simulink model "BicycleHome"  (R2017b)
settings: Solver=VariableStepAuto  StartTime=0.0  StopTime=100  RelTol=1e-3
values from neighbouring files (symbols this model uses):
  b_contact_FW = 2e3    (= 2000)    [BicycleInit.m]
  b_contact_RW = 2e3    (= 2000)    [BicycleInit.m]
  C_F_alpha = 2e4    (= 20000)    [BicycleInit.m]
  C_F_kappa = 2e4    (= 20000)    [BicycleInit.m]
  CM_phi = 1e-1    (= 0.1)    [BicycleInit.m]
  Dtheta0 = -v0 / radiusRW    (= -24.3333333333)    [BicycleInit.m]
  Dtheta0_FW = -v0 / radiusFW    (= -20.8571428571)    [BicycleInit.m]
  epsilon = 1e-2    (= 0.01)    [BicycleInit.m]
  g = 9.81    [BicycleInit.m]
  k_contact_FW = 1e6    (= 1000000)    [BicycleInit.m]
  k_contact_RW = 1e6    (= 1000000)    [BicycleInit.m]
  lengthFF = frontHinge / (sind(lambda))    [BicycleInit.m]
  lengthFW = 0.03    [BicycleInit.m]
  lengthRF = sqrt((w-frontHinge)^2 + adj^2)    [BicycleInit.m]
  lengthRW = 0.03    [BicycleInit.m]
  massFW = 4    [BicycleInit.m]
  massRW = 2    [BicycleInit.m]
  mB = 85    [BicycleInit.m]
  mH = 5    [BicycleInit.m]
  radiusFW = 0.35    [BicycleInit.m]
  radiusRW = 0.3    [BicycleInit.m]
  sigma = 0.12    [BicycleInit.m]
  xPla = 25    [BicycleInit.m]
  yPla = 15    [BicycleInit.m]
  zPla = 0.01    [BicycleInit.m]
undefined symbols (not defined in the file or in its folder): Cylinder, Parts_Lib, sigbuilder_block, X, Y, Z
libraries: nesl_utility x43, sm_lib x37, vrlib x21, dspsrcs4 x2, simulink x2
(part 2 of 3)

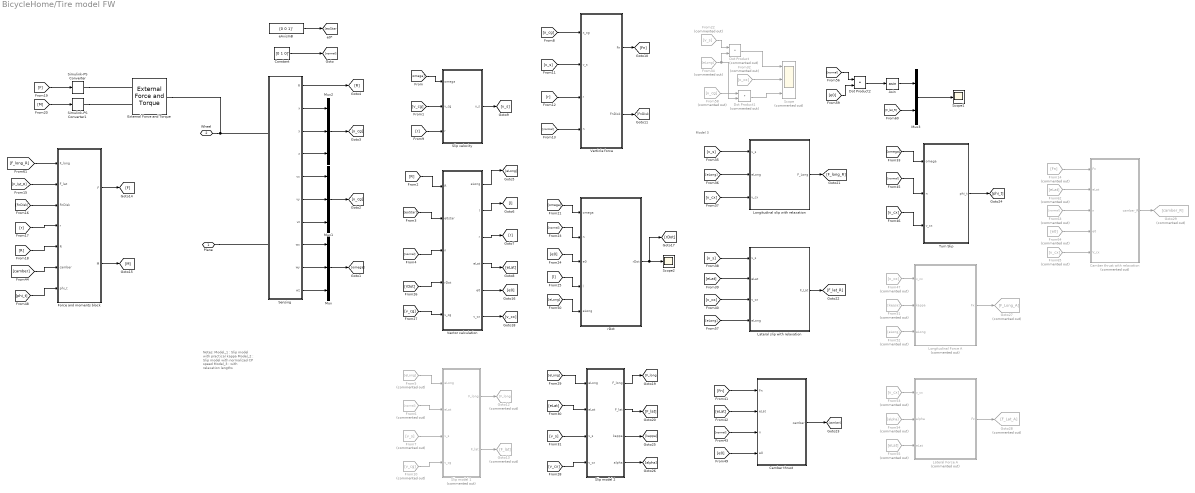
== system BicycleHome/Tire model FW ==
  note: Model 3
  note: Notes:
      | Model_1 : Slip model with practical kappa
      | Model_2 : Slip model with normalized CP speed
      | Model_3 : with relaxation lengths
  Asin : Trigonometry  Operator=asin
  Camber thrust : Subsystem
  Camber thrust with relaxation : Subsystem  Commented=on
  Constant : Constant  Value=[0 1 0]'
  Dot Product : DotProduct  Commented=on  InputSameDT=on  OutDataTypeStr=Inherit: Inherit via internal rule
  Dot Product1 : DotProduct  Commented=on  InputSameDT=on  OutDataTypeStr=Inherit: Inherit via internal rule
  Dot Product2 : DotProduct  InputSameDT=on  OutDataTypeStr=Inherit: Inherit via internal rule
  External Force and Torque : sm_lib/Forces and Torques/External Force and Torque  ForceResolutionFrame=AttachedFrame  EnableForceX=off  EnableForceY=off  EnableForceZ=off  EnableForce=on  TorqueResolutionFrame=AttachedFrame  EnableTorqueX=off  EnableTorqueY=off  EnableTorqueZ=off  EnableTorque=on
  Force and moments block : Subsystem
  From10 : From  Commented=on  GotoTag=v_cg
  From14 : From  Commented=on  GotoTag=Fn
  From22 : From  Commented=on  GotoTag=v_s
  From{32,47,53,65} (4 alike) : From  Commented=on  GotoTag=v_cx
  From34 : From  Commented=on  GotoTag=eLong
  From5 : From  Commented=on  GotoTag=eLong
  From51 : From  Commented=on  GotoTag=kappa
  From52 : From  Commented=on  GotoTag=eLong
  From54 : From  Commented=on  GotoTag=alpha
  From55 : From  Commented=on  GotoTag=eLat
  From58 : From  Commented=on  GotoTag=v_cg
  From6 : From  Commented=on  GotoTag=normal
  From62 : From  Commented=on  GotoTag=eLat
  From63 : From  Commented=on  GotoTag=normal
  From64 : From  Commented=on  GotoTag=e0
  From7 : From  Commented=on  GotoTag=v_s
  Goto12 : Goto  Commented=on  GotoTag=F_long
  Goto13 : Goto  Commented=on  GotoTag=F_lat
  Goto27 : Goto  Commented=on  GotoTag=F_Long_A
  Goto28 : Goto  Commented=on  GotoTag=F_Lat_A
  Goto29 : Goto  Commented=on  GotoTag=camber_R
  Lateral Force A : Subsystem  Commented=on
  Lateral slip with relaxation : Subsystem
  Longitudinal Force A : Subsystem  Commented=on
  Longitudinal slip with relaxation : Subsystem
  Mux : Mux  Inputs=3
  Mux1 : Mux  Inputs=3
  Mux2 : Mux  Inputs=3
  Mux3 : Mux  Inputs=2
  Scope : Scope  Commented=on  NumInputPorts=3
  Scope1 : Scope
  Scope2 : Scope
  Sensing : Subsystem
  Simulink-PS Converter : nesl_utility/Simulink-PS Converter  PhysicalDomain=network_engine_domain  SubClassName=ps_input  LeftPortType=input  RightPortType=output  PseudoPeriodic=off  Frequencies=[]  NoiseDistribution=none  NoiseParameters=[]  Unit=N  AffineConversion=off  FilteringAndDerivatives=provide  SimscapeFilterOrder=1  InputFilterTimeConstant=0.001  UdotUserProvided=0
  Simulink-PS Converter1 : nesl_utility/Simulink-PS Converter  PhysicalDomain=network_engine_domain  SubClassName=ps_input  LeftPortType=input  RightPortType=output  PseudoPeriodic=off  Frequencies=[]  NoiseDistribution=none  NoiseParameters=[]  Unit=N*m  AffineConversion=off  FilteringAndDerivatives=provide  SimscapeFilterOrder=1  InputFilterTimeConstant=0.001  UdotUserProvided=0
  Slip model 1 : Subsystem  Commented=on
  Slip model 2 : Subsystem
  Slip velocity : Subsystem
  Turn Slip : Subsystem
  Vector calculation : Subsystem
  Verticle force : Subsystem
  eAxisInB : Constant  Value=[0 0 1]'
  rDot : Subsystem
  Plane : PMIOPort  Port=1  Side=Left
  Wheel : PMIOPort  Port=2  Side=Right
  wires:
  eAxisInB/1 -> [eoStar]
  Constant/1 -> [normal]
  Sensing/8(wx) -> Mux/1
  Sensing/9(wy) -> Mux/2
  Sensing/10(wz) -> Mux/3
  Mux/1 -> [omega]
  [omega] -> Slip velocity/1(omega)
  Sensing/5(vx) -> Mux1/1
  Sensing/6(vy) -> Mux1/2
  Sensing/7(vz) -> Mux1/3
  Mux1/1 -> [v_cg]
  [v_cg] -> Slip velocity/2(v_cg)
  Sensing/2(x) -> Mux2/1
  Sensing/3(y) -> Mux2/2
  Sensing/4(z) -> Mux2/3
  Mux2/1 -> [x_cg]
  Sensing/1(R) -> [R]
  [R] -> Vector calculation/1(R)
  [eoStar] -> Vector calculation/2(e0star)
  [normal] -> Vector calculation/3(n)
  From5/1 -> Slip model 1/1(eLong)
  From6/1 -> Slip model 1/2(eLat)
  Vector calculation/1(eLong) -> [eLong]
  Vector calculation/2(l) -> [l]
  Vector calculation/3(r) -> [r]
  Vector calculation/4(eLat) -> [eLat]
  [r] -> Slip velocity/3(r)
  Slip velocity/1(v_s) -> [v_s]
  From7/1 -> Slip model 1/3(v_s)
  From10/1 -> Slip model 1/4(v_cg)
  [x_cg] -> Verticle force/1(x_cg)
  [v_s] -> Verticle force/2(v_s)
  [r] -> Verticle force/3(r)
  [normal] -> Verticle force/4(n)
  Verticle force/1(Fn) -> [Fn]
  Verticle force/2(FnDisk) -> [FnDisk]
  Slip model 1/1(F_long) -> Goto12/1
  Slip model 1/2(F_lat) -> Goto13/1
  [r] -> Force and moments block/4(r)
  [R] -> Force and moments block/5(R)
  [F] -> Simulink-PS Converter/1
  [M] -> Simulink-PS Converter1/1
  Vector calculation/5(e0) -> [e0]
  [v_cg] -> Vector calculation/5(v_cg)
  Vector calculation/6(v_cx) -> [v_cx]
  Slip model 2/1(F_long) -> [F_long]
  [v_s] -> Slip model 2/3(v_s)
  [eLat] -> Slip model 2/2(eLat)
  [eLong] -> Slip model 2/1(eLong)
  Slip model 2/2(F_lat) -> [F_lat]
  [v_cx] -> Slip model 2/4(v_cx)
  From22/1 -> Dot Product/1
  From34/1 -> Dot Product1/2, Dot Product/2
  Dot Product/1 -> Scope/1
  [v_s] -> Longitudinal slip with relaxation/1(v_s)
  [eLong] -> Longitudinal slip with relaxation/2(eLong)
  [v_cx] -> Longitudinal slip with relaxation/3(v_cx)
  Longitudinal slip with relaxation/1(F_Long) -> [F_long_R]
  [eLat] -> Lateral slip with relaxation/2(eLat)
  Lateral slip with relaxation/1(F_Lat) -> [F_lat_R]
  [v_cx] -> Lateral slip with relaxation/3(v_cx)
  [v_s] -> Lateral slip with relaxation/1(v_s)
  [Fn] -> Camber thrust/1(Fn)
  [eLat] -> Camber thrust/2(eLat)
  [normal] -> Camber thrust/3(n)
  Camber thrust/1(camber) -> [camber]
  [e0] -> Camber thrust/4(e0)
  Force and moments block/1(F) -> [F]
  Force and moments block/2(M) -> [M]
  [eLong] -> Lateral slip with relaxation/4(eLong)
  From32/1 -> Scope/2
  From58/1 -> Dot Product1/1
  Dot Product1/1 -> Scope/3
  [omega] -> rDot/1(omega)
  [normal] -> rDot/2(n)
  [e0] -> rDot/3(e0)
  [l] -> rDot/4(l)
  [eLong] -> rDot/5(eLong)
  rDot/1(rDot) -> [rDot], Scope2/1
  [rDot] -> Vector calculation/4(rDot)
  Slip model 2/3(kappa) -> [kappa]
  [omega] -> Turn Slip/1(omega)
  [normal] -> Turn Slip/2(n)
  [v_cx] -> Turn Slip/3(v_cx)
  Turn Slip/1(phi_t) -> [phi_t]
  From47/1 -> Longitudinal Force A/1(v_cx)
  Slip model 2/4(alpha) -> [alpha]
  From51/1 -> Longitudinal Force A/2(kappa)
  From52/1 -> Longitudinal Force A/3(eLong)
  Longitudinal Force A/1(Fx) -> Goto27/1
  From53/1 -> Lateral Force A/1(v_cx)
  From54/1 -> Lateral Force A/2(alpha)
  From55/1 -> Lateral Force A/3(eLat)
  Lateral Force A/1(Fz) -> Goto28/1
  [normal] -> Dot Product2/1
  [e0] -> Dot Product2/2
  Dot Product2/1 -> Asin/1
  Asin/1 -> Mux3/1
  [F_lat_R] -> Mux3/2
  Mux3/1 -> Scope1/1
  [FnDisk] -> Force and moments block/3(FnDisk)
  [camber] -> Force and moments block/6(camber)
  [F_long_R] -> Force and moments block/1(F_long)
  [F_lat_R] -> Force and moments block/2(F_lat)
  From62/1 -> Camber thrust with relaxation/2(eLat)
  From64/1 -> Camber thrust with relaxation/4(e0)
  From63/1 -> Camber thrust with relaxation/3(n)
  From14/1 -> Camber thrust with relaxation/1(Fn)
  From65/1 -> Camber thrust with relaxation/5(V_cx)
  Camber thrust with relaxation/1(camber_R) -> Goto29/1
  [phi_t] -> Force and moments block/7(phi_t)
  connections:
  Plane/RConn1 -- Sensing/LConn2
  Wheel/RConn1 -- External Force and Torque/RConn1 -- Sensing/LConn1
  Simulink-PS Converter/RConn1 -- External Force and Torque/LConn1
  Simulink-PS Converter1/RConn1 -- External Force and Torque/LConn2

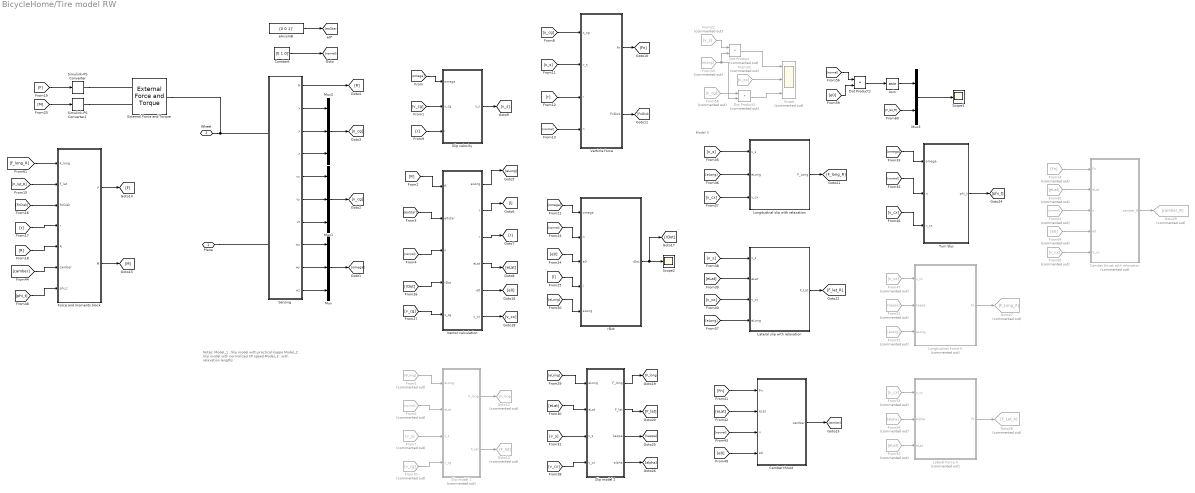
== system BicycleHome/Tire model RW ==
  note: Model 3
  note: Notes:
      | Model_1 : Slip model with practical kappa
      | Model_2 : Slip model with normalized CP speed
      | Model_3 : with relaxation lengths
  Asin : Trigonometry  Operator=asin
  Camber thrust : Subsystem
  Camber thrust with relaxation : Subsystem  Commented=on
  Constant : Constant  Value=[0 1 0]'
  Dot Product : DotProduct  Commented=on  InputSameDT=on  OutDataTypeStr=Inherit: Inherit via internal rule
  Dot Product1 : DotProduct  Commented=on  InputSameDT=on  OutDataTypeStr=Inherit: Inherit via internal rule
  Dot Product2 : DotProduct  InputSameDT=on  OutDataTypeStr=Inherit: Inherit via internal rule
  External Force and Torque : sm_lib/Forces and Torques/External Force and Torque  ForceResolutionFrame=AttachedFrame  EnableForceX=off  EnableForceY=off  EnableForceZ=off  EnableForce=on  TorqueResolutionFrame=AttachedFrame  EnableTorqueX=off  EnableTorqueY=off  EnableTorqueZ=off  EnableTorque=on
  Force and moments block : Subsystem
  From10 : From  Commented=on  GotoTag=v_cg
  From14 : From  Commented=on  GotoTag=Fn
  From22 : From  Commented=on  GotoTag=v_s
  From{32,47,53,65} (4 alike) : From  Commented=on  GotoTag=v_cx
  From34 : From  Commented=on  GotoTag=eLong
  From5 : From  Commented=on  GotoTag=eLong
  From51 : From  Commented=on  GotoTag=kappa
  From52 : From  Commented=on  GotoTag=eLong
  From54 : From  Commented=on  GotoTag=alpha
  From55 : From  Commented=on  GotoTag=eLat
  From58 : From  Commented=on  GotoTag=v_cg
  From6 : From  Commented=on  GotoTag=normal
  From62 : From  Commented=on  GotoTag=eLat
  From63 : From  Commented=on  GotoTag=normal
  From64 : From  Commented=on  GotoTag=e0
  From7 : From  Commented=on  GotoTag=v_s
  Goto12 : Goto  Commented=on  GotoTag=F_long
  Goto13 : Goto  Commented=on  GotoTag=F_lat
  Goto27 : Goto  Commented=on  GotoTag=F_Long_A
  Goto28 : Goto  Commented=on  GotoTag=F_Lat_A
  Goto29 : Goto  Commented=on  GotoTag=camber_R
  Lateral Force A : Subsystem  Commented=on
  Lateral slip with relaxation : Subsystem
  Longitudinal Force A : Subsystem  Commented=on
  Longitudinal slip with relaxation : Subsystem
  Mux : Mux  Inputs=3
  Mux1 : Mux  Inputs=3
  Mux2 : Mux  Inputs=3
  Mux3 : Mux  Inputs=2
  Scope : Scope  Commented=on  NumInputPorts=3
  Scope1 : Scope
  Scope2 : Scope
  Sensing : Subsystem
  Simulink-PS Converter : nesl_utility/Simulink-PS Converter  PhysicalDomain=network_engine_domain  SubClassName=ps_input  LeftPortType=input  RightPortType=output  PseudoPeriodic=off  Frequencies=[]  NoiseDistribution=none  NoiseParameters=[]  Unit=N  AffineConversion=off  FilteringAndDerivatives=provide  SimscapeFilterOrder=1  InputFilterTimeConstant=0.001  UdotUserProvided=0
  Simulink-PS Converter1 : nesl_utility/Simulink-PS Converter  PhysicalDomain=network_engine_domain  SubClassName=ps_input  LeftPortType=input  RightPortType=output  PseudoPeriodic=off  Frequencies=[]  NoiseDistribution=none  NoiseParameters=[]  Unit=N*m  AffineConversion=off  FilteringAndDerivatives=provide  SimscapeFilterOrder=1  InputFilterTimeConstant=0.001  UdotUserProvided=0
  Slip model 1 : Subsystem  Commented=on
  Slip model 2 : Subsystem
  Slip velocity : Subsystem
  Turn Slip : Subsystem
  Vector calculation : Subsystem
  Verticle force : Subsystem
  eAxisInB : Constant  Value=[0 0 1]'
  rDot : Subsystem
  Plane : PMIOPort  Port=1  Side=Left
  Wheel : PMIOPort  Port=2  Side=Right
  wires:
  eAxisInB/1 -> [eoStar]
  Constant/1 -> [normal]
  Sensing/8(wx) -> Mux/1
  Sensing/9(wy) -> Mux/2
  Sensing/10(wz) -> Mux/3
  Mux/1 -> [omega]
  [omega] -> Slip velocity/1(omega)
  Sensing/5(vx) -> Mux1/1
  Sensing/6(vy) -> Mux1/2
  Sensing/7(vz) -> Mux1/3
  Mux1/1 -> [v_cg]
  [v_cg] -> Slip velocity/2(v_cg)
  Sensing/2(x) -> Mux2/1
  Sensing/3(y) -> Mux2/2
  Sensing/4(z) -> Mux2/3
  Mux2/1 -> [x_cg]
  Sensing/1(R) -> [R]
  [R] -> Vector calculation/1(R)
  [eoStar] -> Vector calculation/2(e0star)
  [normal] -> Vector calculation/3(n)
  From5/1 -> Slip model 1/1(eLong)
  From6/1 -> Slip model 1/2(eLat)
  Vector calculation/1(eLong) -> [eLong]
  Vector calculation/2(l) -> [l]
  Vector calculation/3(r) -> [r]
  Vector calculation/4(eLat) -> [eLat]
  [r] -> Slip velocity/3(r)
  Slip velocity/1(v_s) -> [v_s]
  From7/1 -> Slip model 1/3(v_s)
  From10/1 -> Slip model 1/4(v_cg)
  [x_cg] -> Verticle force/1(x_cg)
  [v_s] -> Verticle force/2(v_s)
  [r] -> Verticle force/3(r)
  [normal] -> Verticle force/4(n)
  Verticle force/1(Fn) -> [Fn]
  Verticle force/2(FnDisk) -> [FnDisk]
  Slip model 1/1(F_long) -> Goto12/1
  Slip model 1/2(F_lat) -> Goto13/1
  [r] -> Force and moments block/4(r)
  [R] -> Force and moments block/5(R)
  [F] -> Simulink-PS Converter/1
  [M] -> Simulink-PS Converter1/1
  Vector calculation/5(e0) -> [e0]
  [v_cg] -> Vector calculation/5(v_cg)
  Vector calculation/6(v_cx) -> [v_cx]
  Slip model 2/1(F_long) -> [F_long]
  [v_s] -> Slip model 2/3(v_s)
  [eLat] -> Slip model 2/2(eLat)
  [eLong] -> Slip model 2/1(eLong)
  Slip model 2/2(F_lat) -> [F_lat]
  [v_cx] -> Slip model 2/4(v_cx)
  From22/1 -> Dot Product/1
  From34/1 -> Dot Product1/2, Dot Product/2
  Dot Product/1 -> Scope/1
  [v_s] -> Longitudinal slip with relaxation/1(v_s)
  [eLong] -> Longitudinal slip with relaxation/2(eLong)
  [v_cx] -> Longitudinal slip with relaxation/3(v_cx)
  Longitudinal slip with relaxation/1(F_Long) -> [F_long_R]
  [eLat] -> Lateral slip with relaxation/2(eLat)
  Lateral slip with relaxation/1(F_Lat) -> [F_lat_R]
  [v_cx] -> Lateral slip with relaxation/3(v_cx)
  [v_s] -> Lateral slip with relaxation/1(v_s)
  [Fn] -> Camber thrust/1(Fn)
  [eLat] -> Camber thrust/2(eLat)
  [normal] -> Camber thrust/3(n)
  Camber thrust/1(camber) -> [camber]
  [e0] -> Camber thrust/4(e0)
  Force and moments block/1(F) -> [F]
  Force and moments block/2(M) -> [M]
  [eLong] -> Lateral slip with relaxation/4(eLong)
  From32/1 -> Scope/2
  From58/1 -> Dot Product1/1
  Dot Product1/1 -> Scope/3
  [omega] -> rDot/1(omega)
  [normal] -> rDot/2(n)
  [e0] -> rDot/3(e0)
  [l] -> rDot/4(l)
  [eLong] -> rDot/5(eLong)
  rDot/1(rDot) -> [rDot], Scope2/1
  [rDot] -> Vector calculation/4(rDot)
  Slip model 2/3(kappa) -> [kappa]
  [omega] -> Turn Slip/1(omega)
  [normal] -> Turn Slip/2(n)
  [v_cx] -> Turn Slip/3(v_cx)
  Turn Slip/1(phi_t) -> [phi_t]
  From47/1 -> Longitudinal Force A/1(v_cx)
  Slip model 2/4(alpha) -> [alpha]
  From51/1 -> Longitudinal Force A/2(kappa)
  From52/1 -> Longitudinal Force A/3(eLong)
  Longitudinal Force A/1(Fx) -> Goto27/1
  From53/1 -> Lateral Force A/1(v_cx)
  From54/1 -> Lateral Force A/2(alpha)
  From55/1 -> Lateral Force A/3(eLat)
  Lateral Force A/1(Fz) -> Goto28/1
  [normal] -> Dot Product2/1
  [e0] -> Dot Product2/2
  Dot Product2/1 -> Asin/1
  Asin/1 -> Mux3/1
  [F_lat_R] -> Mux3/2
  Mux3/1 -> Scope1/1
  [FnDisk] -> Force and moments block/3(FnDisk)
  [camber] -> Force and moments block/6(camber)
  [F_long_R] -> Force and moments block/1(F_long)
  [F_lat_R] -> Force and moments block/2(F_lat)
  From62/1 -> Camber thrust with relaxation/2(eLat)
  From64/1 -> Camber thrust with relaxation/4(e0)
  From63/1 -> Camber thrust with relaxation/3(n)
  From14/1 -> Camber thrust with relaxation/1(Fn)
  From65/1 -> Camber thrust with relaxation/5(V_cx)
  Camber thrust with relaxation/1(camber_R) -> Goto29/1
  [phi_t] -> Force and moments block/7(phi_t)
  connections:
  Plane/RConn1 -- Sensing/LConn2
  Wheel/RConn1 -- External Force and Torque/RConn1 -- Sensing/LConn1
  Simulink-PS Converter/RConn1 -- External Force and Torque/LConn1
  Simulink-PS Converter1/RConn1 -- External Force and Torque/LConn2

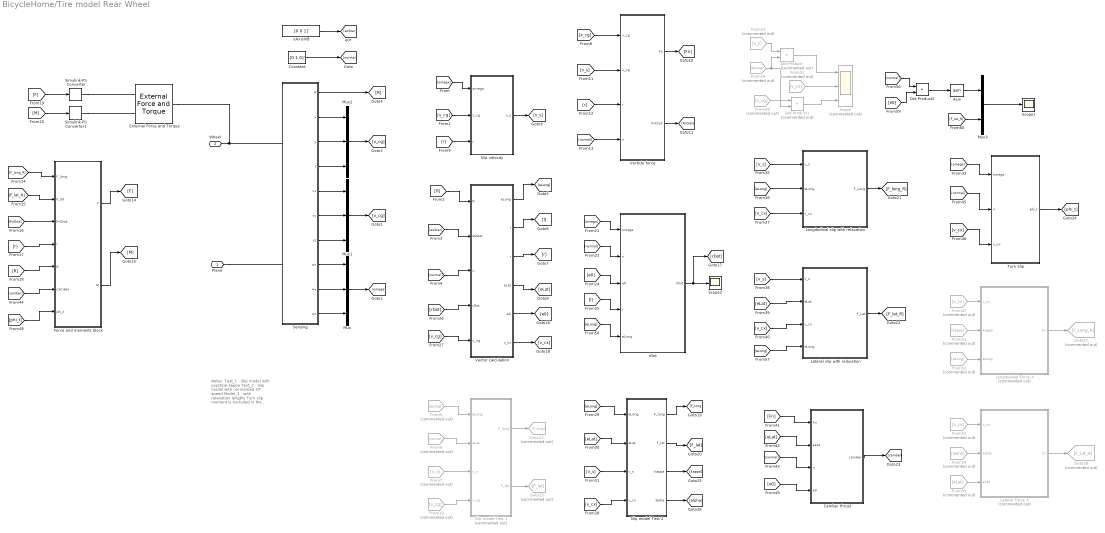
== system BicycleHome/Tire model Rear Wheel ==
  note: Notes:
      | Test_1 : Slip model with practical kappa
      | Test_2 : Slip model with normalized CP speed
      | Model_3 : with relaxation lengths
      |
      | Turn slip moment is excluded in the model as per the
      | paper by RS Sharp
  Asin : Trigonometry  Operator=asin
  Camber thrust : Subsystem
  Constant : Constant  Value=[0 1 0]'
  Dot Product : DotProduct  Commented=on  InputSameDT=on  OutDataTypeStr=Inherit: Inherit via internal rule
  Dot Product1 : DotProduct  Commented=on  InputSameDT=on  OutDataTypeStr=Inherit: Inherit via internal rule
  Dot Product2 : DotProduct  InputSameDT=on  OutDataTypeStr=Inherit: Inherit via internal rule
  External Force and Torque : sm_lib/Forces and Torques/External Force and Torque  ForceResolutionFrame=AttachedFrame  EnableForceX=off  EnableForceY=off  EnableForceZ=off  EnableForce=on  TorqueResolutionFrame=AttachedFrame  EnableTorqueX=off  EnableTorqueY=off  EnableTorqueZ=off  EnableTorque=on
  Force and moments block : Subsystem
  From10 : From  Commented=on  GotoTag=v_cg
  From22 : From  Commented=on  GotoTag=v_s
  From32 : From  Commented=on  GotoTag=v_cx
  From34 : From  Commented=on  GotoTag=eLong
  From47 : From  Commented=on  GotoTag=v_cx
  From5 : From  Commented=on  GotoTag=eLong
  From51 : From  Commented=on  GotoTag=kappa
  From52 : From  Commented=on  GotoTag=eLong
  From53 : From  Commented=on  GotoTag=v_cx
  From54 : From  Commented=on  GotoTag=alpha
  From55 : From  Commented=on  GotoTag=eLat
  From58 : From  Commented=on  GotoTag=v_cg
  From6 : From  Commented=on  GotoTag=normal
  From7 : From  Commented=on  GotoTag=v_s
  Goto12 : Goto  Commented=on  GotoTag=F_long
  Goto13 : Goto  Commented=on  GotoTag=F_lat
  Goto27 : Goto  Commented=on  GotoTag=F_Long_A
  Goto28 : Goto  Commented=on  GotoTag=F_Lat_A
  Lateral Force A : Subsystem  Commented=on
  Lateral slip with relaxation : Subsystem
  Longitudinal Force A : Subsystem  Commented=on
  Longitudinal slip with relaxation : Subsystem
  Mux : Mux  Inputs=3
  Mux1 : Mux  Inputs=3
  Mux2 : Mux  Inputs=3
  Mux3 : Mux  Inputs=2
  Scope : Scope  Commented=on  NumInputPorts=3
  Scope1 : Scope
  Scope2 : Scope
  Sensing : Subsystem
  Simulink-PS Converter : nesl_utility/Simulink-PS Converter  PhysicalDomain=network_engine_domain  SubClassName=ps_input  LeftPortType=input  RightPortType=output  PseudoPeriodic=off  Frequencies=[]  NoiseDistribution=none  NoiseParameters=[]  Unit=N  AffineConversion=off  FilteringAndDerivatives=provide  SimscapeFilterOrder=1  InputFilterTimeConstant=0.001  UdotUserProvided=0
  Simulink-PS Converter1 : nesl_utility/Simulink-PS Converter  PhysicalDomain=network_engine_domain  SubClassName=ps_input  LeftPortType=input  RightPortType=output  PseudoPeriodic=off  Frequencies=[]  NoiseDistribution=none  NoiseParameters=[]  Unit=N*m  AffineConversion=off  FilteringAndDerivatives=provide  SimscapeFilterOrder=1  InputFilterTimeConstant=0.001  UdotUserProvided=0
  Slip model Test 1 : Subsystem  Commented=on
  Slip model Test 2 : Subsystem
  Slip velocity : Subsystem
  Turn Slip : Subsystem
  Vector calculation : Subsystem
  Verticle force : Subsystem
  eAxisInB : Constant  Value=[0 0 1]'
  rDot : Subsystem
  Plane : PMIOPort  Port=1  Side=Left
  Wheel : PMIOPort  Port=2  Side=Right
  wires:
  eAxisInB/1 -> [eoStar]
  Constant/1 -> [normal]
  Sensing/8(wx) -> Mux/1
  Sensing/9(wy) -> Mux/2
  Sensing/10(wz) -> Mux/3
  Mux/1 -> [omega]
  [omega] -> Slip velocity/1(omega)
  Sensing/5(vx) -> Mux1/1
  Sensing/6(vy) -> Mux1/2
  Sensing/7(vz) -> Mux1/3
  Mux1/1 -> [v_cg]
  [v_cg] -> Slip velocity/2(v_cg)
  Sensing/2(x) -> Mux2/1
  Sensing/3(y) -> Mux2/2
  Sensing/4(z) -> Mux2/3
  Mux2/1 -> [x_cg]
  Sensing/1(R) -> [R]
  [R] -> Vector calculation/1(R)
  [eoStar] -> Vector calculation/2(e0star)
  [normal] -> Vector calculation/3(n)
  From5/1 -> Slip model Test 1/1(eLong)
  From6/1 -> Slip model Test 1/2(eLat)
  Vector calculation/1(eLong) -> [eLong]
  Vector calculation/2(l) -> [l]
  Vector calculation/3(r) -> [r]
  Vector calculation/4(eLat) -> [eLat]
  [r] -> Slip velocity/3(r)
  Slip velocity/1(v_s) -> [v_s]
  From7/1 -> Slip model Test 1/3(v_s)
  From10/1 -> Slip model Test 1/4(v_cg)
  [x_cg] -> Verticle force/1(x_cg)
  [v_s] -> Verticle force/2(v_cg)
  [r] -> Verticle force/3(r)
  [normal] -> Verticle force/4(n)
  Verticle force/1(Fn) -> [Fn]
  Verticle force/2(FnDisk) -> [FnDisk]
  Slip model Test 1/1(F_long) -> Goto12/1
  Slip model Test 1/2(F_lat) -> Goto13/1
  [r] -> Force and moments block/4(r)
  [R] -> Force and moments block/5(R)
  [F] -> Simulink-PS Converter/1
  [M] -> Simulink-PS Converter1/1
  Vector calculation/5(e0) -> [e0]
  [v_cg] -> Vector calculation/5(v_cg)
  Vector calculation/6(v_cx) -> [v_cx]
  Slip model Test 2/1(F_long) -> [F_long]
  [v_s] -> Slip model Test 2/3(v_s)
  [eLat] -> Slip model Test 2/2(eLat)
  [eLong] -> Slip model Test 2/1(eLong)
  Slip model Test 2/2(F_lat) -> [F_lat]
  [v_cx] -> Slip model Test 2/4(v_cx)
  From22/1 -> Dot Product/1
  From34/1 -> Dot Product1/2, Dot Product/2
  Dot Product/1 -> Scope/1
  [v_s] -> Longitudinal slip with relaxation/1(v_s)
  [eLong] -> Longitudinal slip with relaxation/2(eLong)
  [v_cx] -> Longitudinal slip with relaxation/3(v_cx)
  Longitudinal slip with relaxation/1(F_Long) -> [F_long_R]
  [eLat] -> Lateral slip with relaxation/2(eLat)
  Lateral slip with relaxation/1(F_Lat) -> [F_lat_R]
  [v_cx] -> Lateral slip with relaxation/3(v_cx)
  [v_s] -> Lateral slip with relaxation/1(v_s)
  [Fn] -> Camber thrust/1(Fn)
  [eLat] -> Camber thrust/2(eLat)
  [normal] -> Camber thrust/3(n)
  Camber thrust/1(camber) -> [camber]
  [e0] -> Camber thrust/4(e0)
  Force and moments block/1(F) -> [F]
  Force and moments block/2(M) -> [M]
  [eLong] -> Lateral slip with relaxation/4(eLong)
  From32/1 -> Scope/2
  From58/1 -> Dot Product1/1
  Dot Product1/1 -> Scope/3
  [omega] -> rDot/1(omega)
  [normal] -> rDot/2(n)
  [e0] -> rDot/3(e0)
  [l] -> rDot/4(l)
  [eLong] -> rDot/5(eLong)
  rDot/1(rDot) -> [rDot], Scope2/1
  [rDot] -> Vector calculation/4(rDot)
  Slip model Test 2/3(kappa) -> [kappa]
  [omega] -> Turn Slip/1(omega)
  [normal] -> Turn Slip/2(n)
  [v_cx] -> Turn Slip/3(v_cx)
  Turn Slip/1(phi_t) -> [phi_t]
  From47/1 -> Longitudinal Force A/1(v_cx)
  Slip model Test 2/4(alpha) -> [alpha]
  From51/1 -> Longitudinal Force A/2(kappa)
  From52/1 -> Longitudinal Force A/3(eLong)
  Longitudinal Force A/1(Fx) -> Goto27/1
  From53/1 -> Lateral Force A/1(v_cx)
  From54/1 -> Lateral Force A/2(alpha)
  From55/1 -> Lateral Force A/3(eLat)
  Lateral Force A/1(Fz) -> Goto28/1
  [normal] -> Dot Product2/1
  [e0] -> Dot Product2/2
  Dot Product2/1 -> Asin/1
  Asin/1 -> Mux3/1
  [F_lat_R] -> Mux3/2
  Mux3/1 -> Scope1/1
  [FnDisk] -> Force and moments block/3(FnDisk)
  [F_long_R] -> Force and moments block/1(F_long)
  [F_lat_R] -> Force and moments block/2(F_lat)
  [camber] -> Force and moments block/6(camber)
  [phi_t] -> Force and moments block/7(phi_t)
  connections:
  Plane/RConn1 -- Sensing/LConn2
  Wheel/RConn1 -- External Force and Torque/RConn1 -- Sensing/LConn1
  Simulink-PS Converter/RConn1 -- External Force and Torque/LConn1
  Simulink-PS Converter1/RConn1 -- External Force and Torque/LConn2

== system BicycleHome/Tire model FW/Camber thrust ==
  Fn : Inport
  eLat : Inport  Port=2
  n : Inport  Port=3
  e0 : Inport  Port=4
  Dot Product1 : DotProduct  InputSameDT=on  OutDataTypeStr=Inherit: Inherit via internal rule
  Product : Product
  Product1 : Product
  Scope1 : Scope
  camber : Outport
  wires:
  Fn/1 -> Product/1
  Product/1 -> Product1/1
  eLat/1 -> Product1/2
  Product1/1 -> Scope1/1, camber/1
  n/1 -> Dot Product1/1
  e0/1 -> Dot Product1/2
  Dot Product1/1 -> Product/2  "sin_gamma"

== system BicycleHome/Tire model FW/Camber thrust with relaxation ==
  Fn : Inport
  eLat : Inport  Port=2
  n : Inport  Port=3
  e0 : Inport  Port=4
  V_cx : Inport  Port=5
  Dot Product1 : DotProduct  InputSameDT=on  OutDataTypeStr=Inherit: Inherit via internal rule
  Gain : Gain  Gain=1/sigma
  Integrator : Integrator
  Product{,1..3} (4 alike) : Product
  Scope1 : Scope
  Sum : Sum  Inputs=|+-
  camber_R : Outport
  wires:
  eLat/1 -> Product1/2
  Product1/1 -> camber_R/1
  n/1 -> Dot Product1/1
  e0/1 -> Dot Product1/2
  V_cx/1 -> Gain/1
  Dot Product1/1 -> Product2/1  "sin_gamma"
  Gain/1 -> Product3/2, Product2/2
  Product2/1 -> Sum/1
  Sum/1 -> Integrator/1
  Integrator/1 -> Product3/1, Product/2  "gamma_F"
  Product3/1 -> Sum/2
  Fn/1 -> Product/1
  Product/1 -> Scope1/1, Product1/1

== system BicycleHome/Tire model FW/Force and moments block ==
  F_long : Inport
  F_lat : Inport  Port=2
  FnDisk : Inport  Port=3
  r : Inport  Port=4
  R : Inport  Port=5
  camber : Inport  Port=6
  phi_t : Inport  Port=7
  Add : Sum  Inputs=4
  Add1 : Sum
  Cross Product : vrlib/Utilities/Cross Product
      settings: SourceProductBaseCode=VR
  Demux : Demux  Outputs=3
  Demux1 : Demux  Outputs=3
  Product : Product  Inputs=/*  Multiplication=Matrix(*)
  Product1 : Product  Inputs=/*  Multiplication=Matrix(*)
  Scope : Scope  NumInputPorts=3
  Scope1 : Scope  NumInputPorts=3
  Scope2 : Scope
  F : Outport
  M : Outport  Port=2
  wires:
  Add/1 -> Cross Product/2, Product/2
  R/1 -> Product1/1, Product/1
  Demux/3 -> Scope/3  "Mz"
  Demux/2 -> Scope/2  "My"
  Demux/1 -> Scope/1  "Mx"
  Cross Product/1 -> Add1/1
  camber/1 -> Add/4
  Product/1 -> Demux1/1, F/1
  Demux1/3 -> Scope1/3  "Fz"
  Demux1/2 -> Scope1/2  "Fy"
  Demux1/1 -> Scope1/1  "Fx"
  F_long/1 -> Add/2
  F_lat/1 -> Add/3
  Add1/1 -> Product1/2
  Product1/1 -> M/1, Demux/1
  r/1 -> Cross Product/1
  phi_t/1 -> Add1/2
  FnDisk/1 -> Add/1

== system BicycleHome/Tire model FW/Lateral Force A ==
  v_cx : Inport
  alpha : Inport  Port=2
  eLat : Inport  Port=3
  Constant : Constant  Value=sigma
  Constant1 : Constant  Value=sigma
  Gain : Gain  Gain=-C_F_alpha
  Integrator : Integrator
  Product{,1..4} (5 alike) : Product
  Scope : Scope
  Scope1 : Scope
  Sum : Sum  Inputs=|+-
  v_cx1 : InportShadow
  Fz : Outport
  wires:
  alpha/1 -> Scope1/1, Product/1  "input"
  v_cx/1 -> Product1/1
  Product/1 -> Sum/1
  Product1/1 -> Product/2
  Constant/1 -> Product1/2
  Sum/1 -> Integrator/1
  Integrator/1 -> Gain/1, Product2/1  "output"
  v_cx1/1 -> Product3/1
  Constant1/1 -> Product3/2
  Product3/1 -> Product2/2
  Product2/1 -> Sum/2
  Gain/1 -> Product4/1
  eLat/1 -> Product4/2
  Product4/1 -> Scope/1, Fz/1

== system BicycleHome/Tire model FW/Lateral slip with relaxation ==
  v_s : Inport
  eLat : Inport  Port=2
  v_cx : Inport  Port=3
  eLong : Inport  Port=4
  Dot Product : DotProduct  InputSameDT=on  OutDataTypeStr=Inherit: Inherit via internal rule
  Gain : Gain  Gain=1/sigma
  Gain1 : Gain  Gain=-C_F_alpha
  Integrator : Integrator
  MATLAB Function2 : MATLAB Function  Commented=through  TreatAsAtomicUnit=on
  Product : Product
  Product1 : Product
  Scope : Scope
  Scope1 : Scope
  Scope2 : Scope
  Sum : Sum  Inputs=|+-
  F_Lat : Outport
  wires:
  v_s/1 -> Dot Product/1
  eLat/1 -> Product1/2, Dot Product/2
  Product/1 -> Sum/2
  Sum/1 -> Gain/1
  Gain/1 -> Integrator/1
  Integrator/1 -> Scope2/1, Gain1/1, Product/2  "alpha_F"
  Gain1/1 -> Product1/1
  Product1/1 -> Scope/1, F_Lat/1
  v_cx/1 -> Product/1
  Dot Product/1 -> MATLAB Function2/1("s1 ")  "s2"
  MATLAB Function2/1(s1) -> Scope1/1, Sum/1

== system BicycleHome/Tire model FW/Longitudinal Force A ==
  v_cx : Inport
  kappa : Inport  Port=2
  eLong : Inport  Port=3
  Constant : Constant  Value=sigma
  Constant1 : Constant  Value=sigma
  Gain : Gain  Gain=-C_F_kappa
  Integrator : Integrator
  Product{,1..4} (5 alike) : Product
  Scope : Scope
  Scope1 : Scope
  Sum : Sum  Inputs=|+-
  v_cx1 : InportShadow
  Fx : Outport
  wires:
  kappa/1 -> Scope1/1, Product/1  "input"
  v_cx/1 -> Product1/1
  Product/1 -> Sum/1
  Product1/1 -> Product/2
  Constant/1 -> Product1/2
  Sum/1 -> Integrator/1
  Integrator/1 -> Gain/1, Product2/1  "output"
  v_cx1/1 -> Product3/1
  Constant1/1 -> Product3/2
  Product3/1 -> Product2/2
  Product2/1 -> Sum/2
  Gain/1 -> Product4/1
  eLong/1 -> Product4/2
  Product4/1 -> Scope/1, Fx/1

== system BicycleHome/Tire model FW/Longitudinal slip with relaxation ==
  v_s : Inport
  eLong : Inport  Port=2
  v_cx : Inport  Port=3
  Dot Product : DotProduct  InputSameDT=on  OutDataTypeStr=Inherit: Inherit via internal rule
  Gain : Gain  Gain=1/sigma
  Gain1 : Gain  Gain=-C_F_kappa
  Integrator : Integrator
  MATLAB Function2 : MATLAB Function  Commented=through  TreatAsAtomicUnit=on
  Product : Product
  Product1 : Product
  Sum : Sum  Inputs=|+-
  F_Long : Outport
  wires:
  v_s/1 -> Dot Product/1
  eLong/1 -> Product1/2, Dot Product/2
  Dot Product/1 -> MATLAB Function2/1("s1 ")  "s1"
  Product/1 -> Sum/2
  Sum/1 -> Gain/1
  Gain/1 -> Integrator/1
  Integrator/1 -> Gain1/1, Product/2  "kappa_F"
  Gain1/1 -> Product1/1
  Product1/1 -> F_Long/1
  v_cx/1 -> Product/1
  MATLAB Function2/1(s1) -> Sum/1

== system BicycleHome/Tire model FW/Sensing ==
  PS-Simulink Converter{,1..9} (10 alike) : nesl_utility/PS-Simulink Converter  PhysicalDomain=network_engine_domain  SubClassName=ps_output  LeftPortType=input  RightPortType=output  PseudoPeriodic=off  Frequencies=[]  Unit=1  AffineConversion=off
  Transform Sensor : sm_lib/Frames and Transforms/Transform Sensor  MeasurementFrame=Base  SenseAngle=off  SenseAxis=off  SenseAngle1=off  SenseAngle2=off  SenseAngle3=off  SenseQ=off  SenseR=on  SenseOmegaX=on  SenseOmegaY=on  SenseOmegaZ=on  SenseOmega1=off  SenseOmega2=off  SenseOmega3=off  SenseQDot=off  SenseRDot=off  SenseAlphaX=off  SenseAlphaY=off  SenseAlphaZ=off  SenseAlpha1=off  SenseAlpha2=off  SenseAlpha3=off  SenseQDDot=off  SenseRDDot=off  SenseX=on  SenseY=on  SenseZ=on  SenseRad=off  SenseAzim=off  SenseDist=off  SenseInc=off  SenseXDot=on  SenseYDot=on  SenseZDot=on  SenseRadDot=off  SenseAzimDot=off  SenseDistDot=off  SenseIncDot=off  SenseXDDot=off  SenseYDDot=off  SenseZDDot=off  SenseRadDDot=off  SenseAzimDDot=off  SenseDistDDot=off  SenseIncDDot=off
  Wheel : PMIOPort  Port=1  Side=Left
  Plane : PMIOPort  Port=2  Side=Left
  R : Outport
  x : Outport  Port=2
  y : Outport  Port=3
  z : Outport  Port=4
  vx : Outport  Port=5
  vy : Outport  Port=6
  vz : Outport  Port=7
  wx : Outport  Port=8
  wy : Outport  Port=9
  wz : Outport  Port=10
  wires:
  PS-Simulink Converter2/1 -> wy/1
  PS-Simulink Converter8/1 -> vy/1
  PS-Simulink Converter9/1 -> vz/1
  PS-Simulink Converter1/1 -> wx/1
  PS-Simulink Converter4/1 -> x/1
  PS-Simulink Converter7/1 -> vx/1
  PS-Simulink Converter3/1 -> wz/1
  PS-Simulink Converter5/1 -> y/1
  PS-Simulink Converter6/1 -> z/1
  PS-Simulink Converter/1 -> R/1
  connections:
  PS-Simulink Converter1/LConn1 -- Transform Sensor/RConn3
  PS-Simulink Converter4/LConn1 -- Transform Sensor/RConn6
  PS-Simulink Converter3/LConn1 -- Transform Sensor/RConn5
  PS-Simulink Converter9/LConn1 -- Transform Sensor/RConn11
  PS-Simulink Converter2/LConn1 -- Transform Sensor/RConn4
  PS-Simulink Converter6/LConn1 -- Transform Sensor/RConn8
  PS-Simulink Converter/LConn1 -- Transform Sensor/RConn2
  Transform Sensor/LConn1 -- Plane/RConn1
  Transform Sensor/RConn1 -- Wheel/RConn1
  PS-Simulink Converter5/LConn1 -- Transform Sensor/RConn7
  PS-Simulink Converter7/LConn1 -- Transform Sensor/RConn9
  PS-Simulink Converter8/LConn1 -- Transform Sensor/RConn10

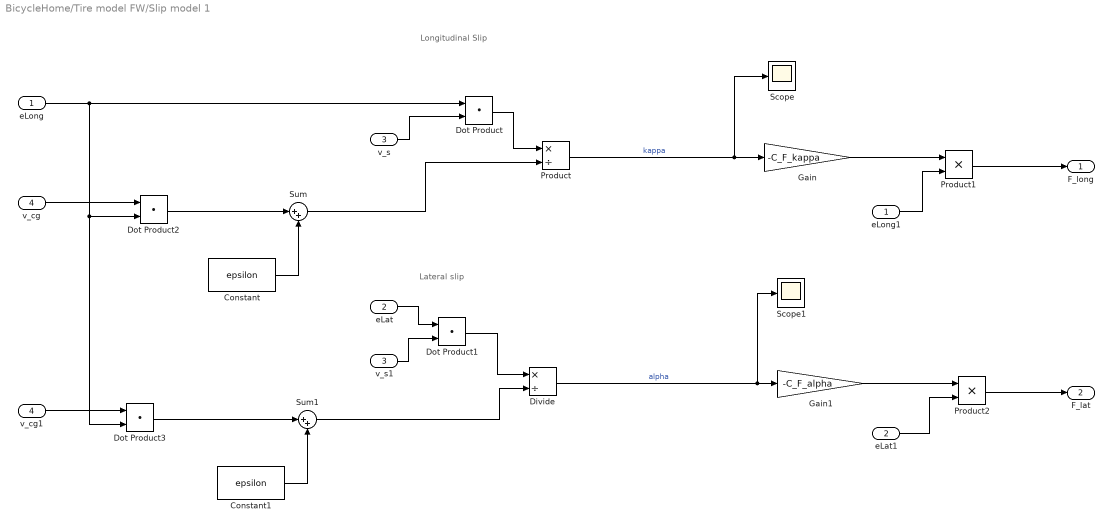
== system BicycleHome/Tire model FW/Slip model 1 ==
  note: Lateral slip
  note: Longitudinal Slip
  eLong : Inport
  eLat : Inport  Port=2
  v_s : Inport  Port=3
  v_cg : Inport  Port=4
  Constant : Constant  Value=epsilon
  Constant1 : Constant  Value=epsilon
  Divide : Product  Inputs=*/
  Dot Product{,1..3} (4 alike) : DotProduct  InputSameDT=on  OutDataTypeStr=Inherit: Inherit via internal rule
  Gain : Gain  Gain=-C_F_kappa
  Gain1 : Gain  Gain=-C_F_alpha
  Product : Product  Inputs=*/
  Product1 : Product
  Product2 : Product
  Scope : Scope
  Scope1 : Scope
  Sum : Sum  Inputs=|++
  Sum1 : Sum  Inputs=|++
  eLat1 : InportShadow  Port=2
  eLong1 : InportShadow
  v_cg1 : InportShadow  Port=4
  v_s1 : InportShadow  Port=3
  F_long : Outport
  F_lat : Outport  Port=2
  wires:
  eLong/1 -> Dot Product3/2, Dot Product2/2, Dot Product/1
  v_s/1 -> Dot Product/2
  Dot Product/1 -> Product/1
  Product/1 -> Scope/1, Gain/1  "kappa"
  eLat/1 -> Dot Product1/1
  v_s1/1 -> Dot Product1/2
  Dot Product1/1 -> Divide/1
  Divide/1 -> Scope1/1, Gain1/1  "alpha"
  Gain/1 -> Product1/1
  eLong1/1 -> Product1/2
  Gain1/1 -> Product2/1
  eLat1/1 -> Product2/2
  Product1/1 -> F_long/1
  Product2/1 -> F_lat/1
  Constant/1 -> Sum/2
  Sum/1 -> Product/2
  Constant1/1 -> Sum1/2
  Sum1/1 -> Divide/2
  v_cg/1 -> Dot Product2/1
  Dot Product2/1 -> Sum/1
  v_cg1/1 -> Dot Product3/1
  Dot Product3/1 -> Sum1/1

== system BicycleHome/Tire model FW/Slip model 2 ==
  note: Lateral slip
  note: Longitudinal Slip
  eLong : Inport
  eLat : Inport  Port=2
  v_s : Inport  Port=3
  v_cx : Inport  Port=4
  Divide : Product  Inputs=*/
  Dot Product : DotProduct  InputSameDT=on  OutDataTypeStr=Inherit: Inherit via internal rule
  Dot Product1 : DotProduct  InputSameDT=on  OutDataTypeStr=Inherit: Inherit via internal rule
  Gain : Gain  Gain=-C_F_kappa
  Gain1 : Gain  Gain=-C_F_alpha
  MATLAB Function1 : MATLAB Function  Commented=through  TreatAsAtomicUnit=on
  MATLAB Function2 : MATLAB Function  Commented=through  TreatAsAtomicUnit=on
  Product : Product  Inputs=*/
  Product1 : Product
  Product2 : Product
  Scope : Scope
  Scope1 : Scope
  eLat1 : InportShadow  Port=2
  eLong1 : InportShadow
  v_cx1 : InportShadow  Port=4
  v_s1 : InportShadow  Port=3
  F_long : Outport
  F_lat : Outport  Port=2
  kappa : Outport  Port=3
  alpha : Outport  Port=4
  wires:
  eLong/1 -> Dot Product/1
  Dot Product/1 -> Product/1
  eLat/1 -> Dot Product1/1
  Dot Product1/1 -> Divide/1
  Divide/1 -> MATLAB Function2/1("s1 ")  "alpha"
  Gain/1 -> Product1/1
  eLong1/1 -> Product1/2
  Gain1/1 -> Product2/1
  eLat1/1 -> Product2/2
  Product1/1 -> F_long/1
  Product2/1 -> F_lat/1
  v_s/1 -> Dot Product/2
  v_s1/1 -> Dot Product1/2
  Product/1 -> MATLAB Function1/1("s1 ")  "kappa"
  v_cx/1 -> Divide/2, Product/2
  MATLAB Function1/1(s1) -> Scope/1, kappa/1, Gain/1
  MATLAB Function2/1(s1) -> alpha/1, Scope1/1, Gain1/1

== system BicycleHome/Tire model FW/Slip velocity ==
  omega : Inport
  v_cg : Inport  Port=2
  r : Inport  Port=3
  Add : Sum
  Cross Product : vrlib/Utilities/Cross Product
      settings: SourceProductBaseCode=VR
  Demux : Demux  Outputs=3
  MATLAB Function1 : MATLAB Function  TreatAsAtomicUnit=on
  MATLAB Function2 : MATLAB Function  TreatAsAtomicUnit=on
  Mux : Mux  Inputs=3
  Scope : Scope
  v_s : Outport
  wires:
  omega/1 -> Cross Product/1
  Cross Product/1 -> Scope/1, Add/2  "v_r"
  r/1 -> Cross Product/2
  v_cg/1 -> Add/1  "V_x"
  Add/1 -> Demux/1
  Demux/1 -> MATLAB Function1/1("s1 ")
  Demux/2 -> Mux/2
  Demux/3 -> MATLAB Function2/1("s1 ")
  MATLAB Function2/1(s1) -> Mux/3
  MATLAB Function1/1(s1) -> Mux/1
  Mux/1 -> v_s/1

== system BicycleHome/Tire model FW/Turn Slip ==
  omega : Inport
  n : Inport  Port=2
  v_cx : Inport  Port=3
  Dot Product : DotProduct  InputSameDT=on  OutDataTypeStr=Inherit: Inherit via internal rule
  Gain : Gain  Gain=1/sigma
  Gain1 : Gain  Gain=-CM_phi
  Gain2 : Gain  Gain=-1
  Integrator : Integrator
  Product : Product
  Product1 : Product
  Product2 : Product  Inputs=*/
  Scope : Scope
  Scope1 : Scope
  Sum : Sum  Inputs=|+-
  phi_t : Outport
  wires:
  omega/1 -> Dot Product/1
  n/1 -> Product/2, Dot Product/2
  Dot Product/1 -> Gain2/1, Sum/1
  Sum/1 -> Gain/1
  Gain/1 -> Integrator/1
  Integrator/1 -> Product1/2, Gain1/1
  Gain1/1 -> Scope/1, Product/1
  Product/1 -> phi_t/1
  v_cx/1 -> Product2/2, Product1/1
  Product1/1 -> Sum/2
  Product2/1 -> Scope1/1
  Gain2/1 -> Product2/1

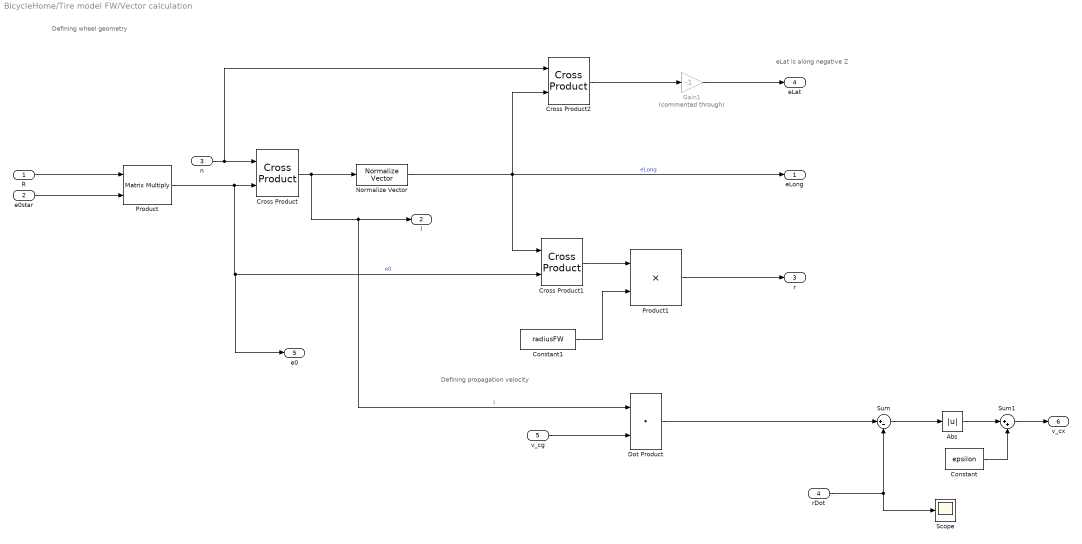
== system BicycleHome/Tire model FW/Vector calculation ==
  note: Defining propagation velocity
  note: Defining wheel geometry
  note: eLat is along
      | negative Z
  R : Inport
  e0star : Inport  Port=2
  n : Inport  Port=3
  rDot : Inport  Port=4
  v_cg : Inport  Port=5
  Abs : Abs  ZeroCross=off
  Constant : Constant  Value=epsilon
  Constant1 : Constant  Value=radiusFW
  Cross Product : vrlib/Utilities/Cross Product
      settings: SourceProductBaseCode=VR
  Cross Product1 : vrlib/Utilities/Cross Product
      settings: SourceProductBaseCode=VR
  Cross Product2 : vrlib/Utilities/Cross Product
      settings: SourceProductBaseCode=VR
  Dot Product : DotProduct  InputSameDT=on  OutDataTypeStr=Inherit: Inherit via internal rule
  Gain1 : Gain  Commented=through  Gain=-1
  Normalize Vector : vrlib/Utilities/Normalize Vector  maxzero=0
      settings: SourceProductName=Simulink 3D Animation  SourceProductBaseCode=VR
  Product : Product  Multiplication=Matrix(*)
  Product1 : Product
  Scope : Scope
  Sum : Sum  Inputs=|+-
  Sum1 : Sum  Inputs=|++
  eLong : Outport
  l : Outport  Port=2
  r : Outport  Port=3
  eLat : Outport  Port=4
  e0 : Outport  Port=5
  v_cx : Outport  Port=6
  wires:
  R/1 -> Product/1
  e0star/1 -> Product/2
  Product/1 -> Cross Product1/2, e0/1, Cross Product/2  "e0"
  n/1 -> Cross Product2/1, Cross Product/1
  Cross Product/1 -> Dot Product/1, l/1, Normalize Vector/1  "l"
  Normalize Vector/1 -> eLong/1, Cross Product2/2, Cross Product1/1  "eLong"
  Cross Product1/1 -> Product1/1
  Cross Product2/1 -> Gain1/1
  v_cg/1 -> Dot Product/2
  Dot Product/1 -> Sum/1
  Sum/1 -> Abs/1
  Abs/1 -> Sum1/1
  Sum1/1 -> v_cx/1
  Constant/1 -> Sum1/2
  Product1/1 -> r/1
  Gain1/1 -> eLat/1
  Constant1/1 -> Product1/2
  rDot/1 -> Sum/2, Scope/1

== system BicycleHome/Tire model FW/Verticle force ==
  x_cg : Inport
  v_s : Inport  Port=2
  r : Inport  Port=3
  n : Inport  Port=4
  Dot Product : DotProduct  InputSameDT=on  OutDataTypeStr=Inherit: Inherit via internal rule
  Dot Product1 : DotProduct  InputSameDT=on  OutDataTypeStr=Inherit: Inherit via internal rule
  Gain : Gain  Gain=-k_contact_FW
  Gain1 : Gain  Gain=-b_contact_FW
  Gain2 : Gain  Commented=through  Gain=-1
  Initial position of CP from ground : Constant  Value=[0 0 0]'
  Product : Product
  Scope : Scope
  Scope1 : Scope
  Sum : Sum  Inputs=|++
  Sum1 : Sum  Inputs=|+-
  Sum2 : Sum
  Fn : Outport
  FnDisk : Outport  Port=2
  wires:
  x_cg/1 -> Sum/1
  Sum/1 -> Scope/1, Sum1/1  "CP position from ground"
  Initial position of CP from ground/1 -> Sum1/2
  Sum1/1 -> Dot Product/1
  v_s/1 -> Dot Product1/2
  Dot Product1/1 -> Gain1/1  "pentration velocity"
  Sum2/1 -> Fn/1, Gain2/1, Scope1/1
  n/1 -> Product/2, Dot Product1/1, Dot Product/2
  r/1 -> Sum/2
  Gain2/1 -> Product/1
  Gain/1 -> Sum2/1
  Dot Product/1 -> Gain/1  "pen"
  Gain1/1 -> Sum2/2
  Product/1 -> FnDisk/1

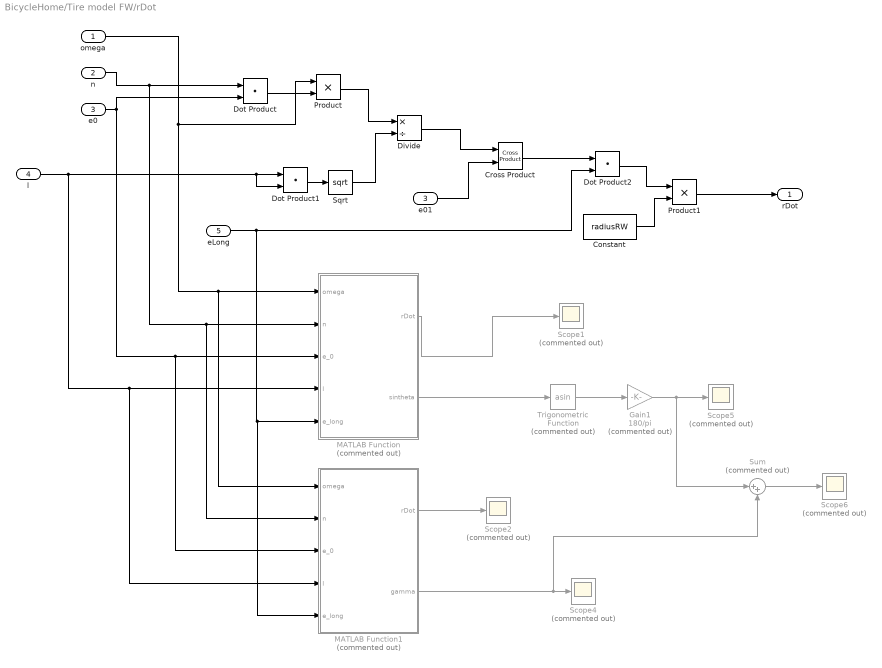
== system BicycleHome/Tire model FW/rDot ==
  omega : Inport
  n : Inport  Port=2
  e0 : Inport  Port=3
  l : Inport  Port=4
  eLong : Inport  Port=5
  Constant : Constant  Value=radiusRW
  Cross Product : vrlib/Utilities/Cross Product
      settings: SourceProductBaseCode=VR
  Divide : Product  Inputs=*/
  Dot Product : DotProduct  InputSameDT=on  OutDataTypeStr=Inherit: Inherit via internal rule
  Dot Product1 : DotProduct  InputSameDT=on  OutDataTypeStr=Inherit: Inherit via internal rule
  Dot Product2 : DotProduct  InputSameDT=on  OutDataTypeStr=Inherit: Inherit via internal rule
  Gain1 : Gain  Commented=on  Gain=180/pi
  MATLAB Function : MATLAB Function  Commented=on  TreatAsAtomicUnit=on
  MATLAB Function1 : MATLAB Function  Commented=on  TreatAsAtomicUnit=on
  Product : Product
  Product1 : Product
  Scope{1..2,4..6} (5 alike) : Scope  Commented=on
  Sqrt : Sqrt  SaturateOnIntegerOverflow=on
  Sum : Sum  Commented=on  Inputs=|++
  Trigonometric Function : Trigonometry  Commented=on  Operator=asin
  e01 : InportShadow  Port=3
  rDot : Outport
  wires:
  n/1 -> MATLAB Function1/2(n), MATLAB Function/2(n), Dot Product/1
  e0/1 -> MATLAB Function1/3(e_0), MATLAB Function/3(e_0), Dot Product/2
  Dot Product/1 -> Product/2
  omega/1 -> MATLAB Function1/1(omega), MATLAB Function/1(omega), Product/1
  Product/1 -> Divide/1
  l/1 -> MATLAB Function1/4(l), MATLAB Function/4(l), Dot Product1/2, Dot Product1/1
  Dot Product1/1 -> Sqrt/1
  Sqrt/1 -> Divide/2
  Divide/1 -> Cross Product/1
  e01/1 -> Cross Product/2
  Cross Product/1 -> Dot Product2/1
  eLong/1 -> MATLAB Function1/5(e_long), MATLAB Function/5(e_long), Dot Product2/2
  Dot Product2/1 -> Product1/1
  Constant/1 -> Product1/2
  MATLAB Function/1(rDot) -> Scope1/1
  MATLAB Function1/1(rDot) -> Scope2/1
  Product1/1 -> rDot/1
  MATLAB Function1/2(gamma) -> Sum/2, Scope4/1
  MATLAB Function/2(sintheta) -> Trigonometric Function/1
  Trigonometric Function/1 -> Gain1/1
  Gain1/1 -> Sum/1, Scope5/1
  Sum/1 -> Scope6/1

== system BicycleHome/Tire model RW/Camber thrust ==
  Fn : Inport
  eLat : Inport  Port=2
  n : Inport  Port=3
  e0 : Inport  Port=4
  Abs : Abs
  Compare To Constant : simulink/Logic and Bit Operations/Compare To Constant  relop=>=  const=1.0  OutDataTypeStr=boolean
  Dot Product1 : DotProduct  InputSameDT=on  OutDataTypeStr=Inherit: Inherit via internal rule
  Gain : Gain  Gain=180/pi
  Product : Product
  Product1 : Product
  Stop Simulation : Stop
  camber : Outport
  tag scope: lean_RW=global
  wires:
  Fn/1 -> Product/1
  Product/1 -> Product1/1
  eLat/1 -> Product1/2
  Product1/1 -> camber/1
  Dot Product1/1 -> Gain/1, Abs/1, Product/2  "sin_gamma"
  n/1 -> Dot Product1/1
  e0/1 -> Dot Product1/2
  Abs/1 -> Compare To Constant/1
  Compare To Constant/1 -> Stop Simulation/1
  Gain/1 -> [lean_RW]

== system BicycleHome/Tire model RW/Camber thrust with relaxation ==
  Fn : Inport
  eLat : Inport  Port=2
  n : Inport  Port=3
  e0 : Inport  Port=4
  V_cx : Inport  Port=5
  Dot Product1 : DotProduct  InputSameDT=on  OutDataTypeStr=Inherit: Inherit via internal rule
  Gain : Gain  Gain=1/sigma
  Integrator : Integrator
  Product{,1..3} (4 alike) : Product
  Scope1 : Scope
  Sum : Sum  Inputs=|+-
  camber_R : Outport
  wires:
  eLat/1 -> Product1/2
  Product1/1 -> camber_R/1
  n/1 -> Dot Product1/1
  e0/1 -> Dot Product1/2
  V_cx/1 -> Gain/1
  Dot Product1/1 -> Product2/1  "sin_gamma"
  Gain/1 -> Product3/2, Product2/2
  Product2/1 -> Sum/1
  Sum/1 -> Integrator/1
  Integrator/1 -> Product3/1, Product/2  "gamma_F"
  Product3/1 -> Sum/2
  Fn/1 -> Product/1
  Product/1 -> Scope1/1, Product1/1

== system BicycleHome/Tire model RW/Force and moments block ==
  F_long : Inport
  F_lat : Inport  Port=2
  FnDisk : Inport  Port=3
  r : Inport  Port=4
  R : Inport  Port=5
  camber : Inport  Port=6
  phi_t : Inport  Port=7
  Add : Sum  Inputs=4
  Add1 : Sum
  Cross Product : vrlib/Utilities/Cross Product
      settings: SourceProductBaseCode=VR
  Demux : Demux  Outputs=3
  Demux1 : Demux  Outputs=3
  Product : Product  Inputs=/*  Multiplication=Matrix(*)
  Product1 : Product  Inputs=/*  Multiplication=Matrix(*)
  Scope : Scope  NumInputPorts=3
  Scope1 : Scope  NumInputPorts=3
  Scope2 : Scope
  F : Outport
  M : Outport  Port=2
  wires:
  Add/1 -> Cross Product/2, Product/2
  R/1 -> Product1/1, Product/1
  Demux/3 -> Scope/3  "Mz"
  Demux/2 -> Scope/2  "My"
  Demux/1 -> Scope/1  "Mx"
  Cross Product/1 -> Add1/1
  camber/1 -> Add/4
  Product/1 -> Demux1/1, F/1
  Demux1/3 -> Scope1/3  "Fz"
  Demux1/2 -> Scope1/2  "Fy"
  Demux1/1 -> Scope1/1  "Fx"
  F_long/1 -> Add/2
  F_lat/1 -> Add/3
  Add1/1 -> Product1/2
  Product1/1 -> M/1, Demux/1
  r/1 -> Cross Product/1
  phi_t/1 -> Add1/2
  FnDisk/1 -> Add/1

== system BicycleHome/Tire model RW/Lateral Force A ==
  v_cx : Inport
  alpha : Inport  Port=2
  eLat : Inport  Port=3
  Constant : Constant  Value=sigma
  Constant1 : Constant  Value=sigma
  Gain : Gain  Gain=-C_F_alpha
  Integrator : Integrator
  Product{,1..4} (5 alike) : Product
  Scope : Scope
  Scope1 : Scope
  Sum : Sum  Inputs=|+-
  v_cx1 : InportShadow
  Fz : Outport
  wires:
  alpha/1 -> Scope1/1, Product/1  "input"
  v_cx/1 -> Product1/1
  Product/1 -> Sum/1
  Product1/1 -> Product/2
  Constant/1 -> Product1/2
  Sum/1 -> Integrator/1
  Integrator/1 -> Gain/1, Product2/1  "output"
  v_cx1/1 -> Product3/1
  Constant1/1 -> Product3/2
  Product3/1 -> Product2/2
  Product2/1 -> Sum/2
  Gain/1 -> Product4/1
  eLat/1 -> Product4/2
  Product4/1 -> Scope/1, Fz/1

== system BicycleHome/Tire model RW/Lateral slip with relaxation ==
  v_s : Inport
  eLat : Inport  Port=2
  v_cx : Inport  Port=3
  eLong : Inport  Port=4
  Dot Product : DotProduct  InputSameDT=on  OutDataTypeStr=Inherit: Inherit via internal rule
  Gain : Gain  Gain=1/sigma
  Gain1 : Gain  Gain=-C_F_alpha
  Integrator : Integrator
  MATLAB Function2 : MATLAB Function  Commented=through  TreatAsAtomicUnit=on
  Product : Product
  Product1 : Product
  Scope : Scope
  Scope1 : Scope
  Scope2 : Scope
  Sum : Sum  Inputs=|+-
  F_Lat : Outport
  wires:
  v_s/1 -> Dot Product/1
  eLat/1 -> Product1/2, Dot Product/2
  Product/1 -> Sum/2
  Sum/1 -> Gain/1
  Gain/1 -> Integrator/1
  Integrator/1 -> Scope2/1, Gain1/1, Product/2  "alpha_F"
  Gain1/1 -> Product1/1
  Product1/1 -> Scope/1, F_Lat/1
  v_cx/1 -> Product/1
  Dot Product/1 -> MATLAB Function2/1("s1 ")  "s2"
  MATLAB Function2/1(s1) -> Scope1/1, Sum/1

== system BicycleHome/Tire model RW/Longitudinal Force A ==
  v_cx : Inport
  kappa : Inport  Port=2
  eLong : Inport  Port=3
  Constant : Constant  Value=sigma
  Constant1 : Constant  Value=sigma
  Gain : Gain  Gain=-C_F_kappa
  Integrator : Integrator
  Product{,1..4} (5 alike) : Product
  Scope : Scope
  Scope1 : Scope
  Sum : Sum  Inputs=|+-
  v_cx1 : InportShadow
  Fx : Outport
  wires:
  kappa/1 -> Scope1/1, Product/1  "input"
  v_cx/1 -> Product1/1
  Product/1 -> Sum/1
  Product1/1 -> Product/2
  Constant/1 -> Product1/2
  Sum/1 -> Integrator/1
  Integrator/1 -> Gain/1, Product2/1  "output"
  v_cx1/1 -> Product3/1
  Constant1/1 -> Product3/2
  Product3/1 -> Product2/2
  Product2/1 -> Sum/2
  Gain/1 -> Product4/1
  eLong/1 -> Product4/2
  Product4/1 -> Scope/1, Fx/1

== system BicycleHome/Tire model RW/Longitudinal slip with relaxation ==
  v_s : Inport
  eLong : Inport  Port=2
  v_cx : Inport  Port=3
  Dot Product : DotProduct  InputSameDT=on  OutDataTypeStr=Inherit: Inherit via internal rule
  Gain : Gain  Gain=1/sigma
  Gain1 : Gain  Gain=-C_F_kappa
  Integrator : Integrator
  MATLAB Function2 : MATLAB Function  Commented=through  TreatAsAtomicUnit=on
  Product : Product
  Product1 : Product
  Sum : Sum  Inputs=|+-
  F_Long : Outport
  wires:
  v_s/1 -> Dot Product/1
  eLong/1 -> Product1/2, Dot Product/2
  Dot Product/1 -> MATLAB Function2/1("s1 ")  "s1"
  Product/1 -> Sum/2
  Sum/1 -> Gain/1
  Gain/1 -> Integrator/1
  Integrator/1 -> Gain1/1, Product/2  "kappa_F"
  Gain1/1 -> Product1/1
  Product1/1 -> F_Long/1
  v_cx/1 -> Product/1
  MATLAB Function2/1(s1) -> Sum/1

== system BicycleHome/Tire model RW/Sensing ==
  PS-Simulink Converter{,1..9} (10 alike) : nesl_utility/PS-Simulink Converter  PhysicalDomain=network_engine_domain  SubClassName=ps_output  LeftPortType=input  RightPortType=output  PseudoPeriodic=off  Frequencies=[]  Unit=1  AffineConversion=off
  Transform Sensor : sm_lib/Frames and Transforms/Transform Sensor  MeasurementFrame=Base  SenseAngle=off  SenseAxis=off  SenseAngle1=off  SenseAngle2=off  SenseAngle3=off  SenseQ=off  SenseR=on  SenseOmegaX=on  SenseOmegaY=on  SenseOmegaZ=on  SenseOmega1=off  SenseOmega2=off  SenseOmega3=off  SenseQDot=off  SenseRDot=off  SenseAlphaX=off  SenseAlphaY=off  SenseAlphaZ=off  SenseAlpha1=off  SenseAlpha2=off  SenseAlpha3=off  SenseQDDot=off  SenseRDDot=off  SenseX=on  SenseY=on  SenseZ=on  SenseRad=off  SenseAzim=off  SenseDist=off  SenseInc=off  SenseXDot=on  SenseYDot=on  SenseZDot=on  SenseRadDot=off  SenseAzimDot=off  SenseDistDot=off  SenseIncDot=off  SenseXDDot=off  SenseYDDot=off  SenseZDDot=off  SenseRadDDot=off  SenseAzimDDot=off  SenseDistDDot=off  SenseIncDDot=off
  Wheel : PMIOPort  Port=1  Side=Left
  Plane : PMIOPort  Port=2  Side=Left
  R : Outport
  x : Outport  Port=2
  y : Outport  Port=3
  z : Outport  Port=4
  vx : Outport  Port=5
  vy : Outport  Port=6
  vz : Outport  Port=7
  wx : Outport  Port=8
  wy : Outport  Port=9
  wz : Outport  Port=10
  wires:
  PS-Simulink Converter2/1 -> wy/1
  PS-Simulink Converter8/1 -> vy/1
  PS-Simulink Converter9/1 -> vz/1
  PS-Simulink Converter1/1 -> wx/1
  PS-Simulink Converter4/1 -> x/1
  PS-Simulink Converter7/1 -> vx/1
  PS-Simulink Converter3/1 -> wz/1
  PS-Simulink Converter5/1 -> y/1
  PS-Simulink Converter6/1 -> z/1
  PS-Simulink Converter/1 -> R/1
  connections:
  PS-Simulink Converter1/LConn1 -- Transform Sensor/RConn3
  PS-Simulink Converter4/LConn1 -- Transform Sensor/RConn6
  PS-Simulink Converter3/LConn1 -- Transform Sensor/RConn5
  PS-Simulink Converter9/LConn1 -- Transform Sensor/RConn11
  PS-Simulink Converter2/LConn1 -- Transform Sensor/RConn4
  PS-Simulink Converter6/LConn1 -- Transform Sensor/RConn8
  PS-Simulink Converter/LConn1 -- Transform Sensor/RConn2
  Transform Sensor/LConn1 -- Plane/RConn1
  Transform Sensor/RConn1 -- Wheel/RConn1
  PS-Simulink Converter5/LConn1 -- Transform Sensor/RConn7
  PS-Simulink Converter7/LConn1 -- Transform Sensor/RConn9
  PS-Simulink Converter8/LConn1 -- Transform Sensor/RConn10
